simulink model "KUKA_LBR_Simulink_model_flatness_based_control"  (R2017a)
settings: Solver=VariableStepAuto  StartTime=0.0  StopTime=T  RelTol=1e-3
InitFcn:
  | main
values from neighbouring files (symbols this model uses):
  elbowAngle = elbowAngle * pi/180    (= 0)    [KUKA_LBR_init.m]    (also in Untitled2.m)
  KAnaJacNum = [k_ind 0 0 0 0 0 ;                 0  k_ind 0 0 0 0 ;                    0 0 k_ind 0 0 0 ;                      0 0 0 k_ind 0 0 ;                        0 0 0 0 k_ind 0 ;                          0 0 0 0 0 k_ind ;                            ]    [KUKA_LBR_init.m]
  Kuka_LBR_param_simu = Simulink.Parameter(Kuka_LBR_param_simu)    [KUKA_LBR_init.m]
  KUKA_LBR_x0 = [x1_0 x2_0 x3_0 x4_0 x5_0 x6_0 x7_0 x8_0 x9_0 x10_0 x11_0 x12_0 x13_0 x14_0]    [KUKA_LBR_init.m]
  rpyDes = rpyDes * pi/180    [KUKA_LBR_init.m]    (also in Untitled2.m)
  T = 0.5    [KUKA_LBR_init.m]
  vecGlobalConfig = [1; 1; 1]    [KUKA_LBR_init.m]    (also in Untitled2.m = [1, 1, 1])
undefined symbols (not defined in the file or in its folder): Kuka_LBR_param
(part 1 of 19)
settings Model: Creator=pc  LastModifiedBy=pc

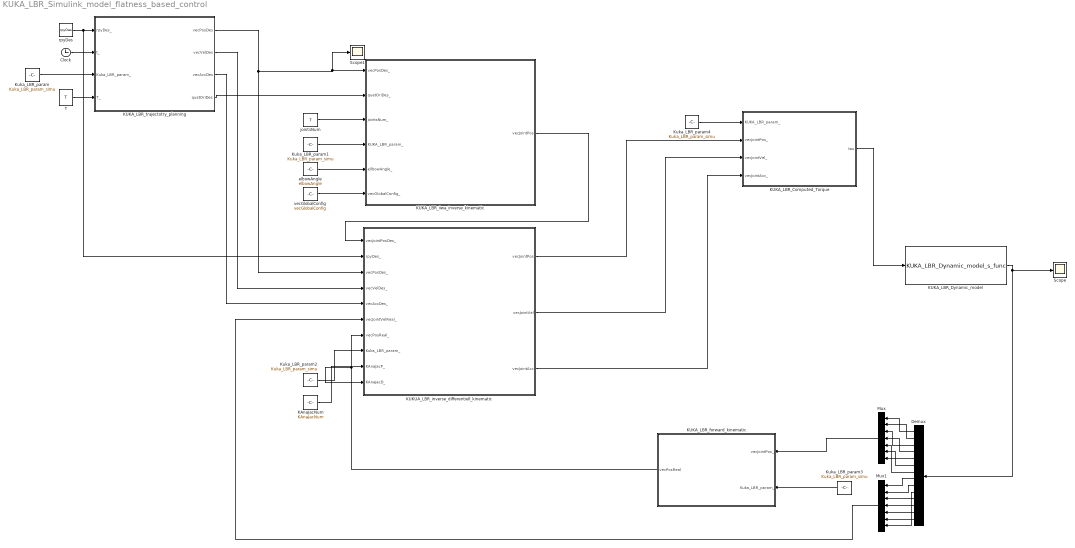
== system KUKA_LBR_Simulink_model_flatness_based_control ==
  Clock : Clock
  Demux : Demux  Outputs=14
  KAnaJacNum : Constant  Value=KAnaJacNum
  KUKA_LBR_Computed_Torque : MATLAB Function  TreatAsAtomicUnit=on
  KUKA_LBR_Dynamic_model : M-S-Function  FunctionName=KUKA_LBR_Dynamic_model_s_func  Parameters=KUKA_LBR_x0,Kuka_LBR_param
  KUKA_LBR_forward_kinematic : MATLAB Function  TreatAsAtomicUnit=on
  KUKA_LBR_iiwa_inverse_kinematic : MATLAB Function  TreatAsAtomicUnit=on
  KUKA_LBR_trajectotry_planning : MATLAB Function  TreatAsAtomicUnit=on
  KUKUA_LBR_inverse_differentiell_kinematic : MATLAB Function  TreatAsAtomicUnit=on
  Kuka_LBR_param{,1..4} (5 alike) : Constant  Value=Kuka_LBR_param_simu  OutDataTypeStr=Bus: Kuka_LBR_param_simu_Type
  Mux : Mux  Inputs=7
  Mux1 : Mux  Inputs=7
  Scope : Scope
  Scope1 : Scope
  T : Constant  Value=T
  elbowAngle : Constant  Value=elbowAngle
  jointsNum : Constant  Value=7
  rpyDes : Constant  Value=rpyDes
  vecGlobalConfig : Constant  Value=vecGlobalConfig
  wires:
  jointsNum/1 -> KUKA_LBR_iiwa_inverse_kinematic/3(jointsNum_)
  elbowAngle/1 -> KUKA_LBR_iiwa_inverse_kinematic/5(ellbowAngle_)
  vecGlobalConfig/1 -> KUKA_LBR_iiwa_inverse_kinematic/6(vecGlobalConfig_)
  KUKUA_LBR_inverse_differentiell_kinematic/2(vecJointVel) -> KUKA_LBR_Computed_Torque/3(vecJointVel_)
  KUKA_LBR_Computed_Torque/1(tau) -> KUKA_LBR_Dynamic_model/1
  KUKA_LBR_iiwa_inverse_kinematic/1(vecJointPos) -> KUKUA_LBR_inverse_differentiell_kinematic/1(vecJointPosDes_)
  KUKA_LBR_Dynamic_model/1 -> Scope/1, Demux/1
  Demux/1 -> Mux/1
  Demux/2 -> Mux/2
  Demux/3 -> Mux/3
  Demux/4 -> Mux/4
  Demux/5 -> Mux/5
  Demux/6 -> Mux/6
  Demux/7 -> Mux/7
  Mux/1 -> KUKA_LBR_forward_kinematic/1(vecJointPos_)
  Demux/8 -> Mux1/1
  Demux/9 -> Mux1/2
  Demux/10 -> Mux1/3
  Demux/11 -> Mux1/4
  Demux/12 -> Mux1/5
  Demux/13 -> Mux1/6
  Demux/14 -> Mux1/7
  Kuka_LBR_param3/1 -> KUKA_LBR_forward_kinematic/2(Kuka_LBR_param_)
  KUKA_LBR_forward_kinematic/1(vecPosReal) -> KUKUA_LBR_inverse_differentiell_kinematic/10(KAnaJacD_), KUKUA_LBR_inverse_differentiell_kinematic/7(vecPosReal_)
  Mux1/1 -> KUKUA_LBR_inverse_differentiell_kinematic/6(vecJointVelReal_)
  KUKUA_LBR_inverse_differentiell_kinematic/3(vecJointAcc) -> KUKA_LBR_Computed_Torque/4(vecJointAcc_)
  KUKA_LBR_trajectotry_planning/1(vecPosDes) -> KUKUA_LBR_inverse_differentiell_kinematic/3(vecPosDes_), Scope1/1, KUKA_LBR_iiwa_inverse_kinematic/1(vecPosDes_)
  KUKA_LBR_trajectotry_planning/4(quatOriDes) -> KUKA_LBR_iiwa_inverse_kinematic/2(quatOriDes_)
  Clock/1 -> KUKA_LBR_trajectotry_planning/2(t_)
  Kuka_LBR_param/1 -> KUKA_LBR_trajectotry_planning/3(Kuka_LBR_param_)
  rpyDes/1 -> KUKUA_LBR_inverse_differentiell_kinematic/2(rpyDes_), KUKA_LBR_trajectotry_planning/1(rpyDes_)
  T/1 -> KUKA_LBR_trajectotry_planning/4(T_)
  KUKA_LBR_trajectotry_planning/2(vecVelDes) -> KUKUA_LBR_inverse_differentiell_kinematic/4(vecVelDes_)
  Kuka_LBR_param4/1 -> KUKA_LBR_Computed_Torque/1(KUKA_LBR_param_)
  Kuka_LBR_param1/1 -> KUKA_LBR_iiwa_inverse_kinematic/4(KUKA_LBR_param_)
  Kuka_LBR_param2/1 -> KUKUA_LBR_inverse_differentiell_kinematic/8(Kuka_LBR_param_)
  KUKUA_LBR_inverse_differentiell_kinematic/1(vecJointPos) -> KUKA_LBR_Computed_Torque/2(vecJointPos_)
  KAnaJacNum/1 -> KUKUA_LBR_inverse_differentiell_kinematic/9(KAnaJacP_)
  KUKA_LBR_trajectotry_planning/3(vecAccDes) -> KUKUA_LBR_inverse_differentiell_kinematic/5(vecAccDes_)
